simulink model "RIP_LQR_OK"  (Simulink 8.1)
settings: Solver=ode45  StartTime=0.0  StopTime=30  RelTol=1e-3
StopFcn:
  | plot(Data.time, Data.signals(1,1).values,'-r', 'LineWidth', 1.5)
  | hold on;
  | plot(Data.time, Data.signals(1,2).values,'-b', 'LineWidth',1.5)
  | grid;
  | legend('alpha','theta');
  | 
  | ylabel('alpha, theta [deg]');
libraries: aerolibconvert2 x4
settings Model: Creator=ThanhNhan  LastModifiedBy=ThanhNhan
settings DataIOCC: SignalLoggingSaveFormat=Dataset
settings OptimizationCC: ExpressionDepthLimit=128
settings DebuggingCC: FcnCallInpInsideContextMsg=EnableAllAsError
settings GRTTargetCC: CombineOutputUpdateFcns=on  GRTInterface=off

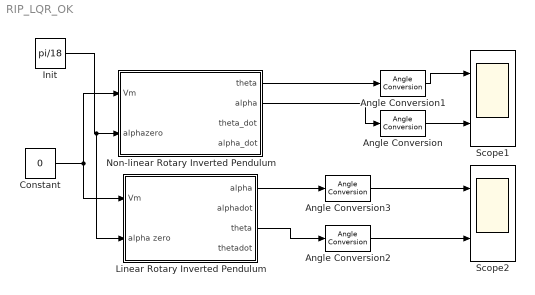
== system RIP_LQR_OK ==
  Angle Conversion{,1..3} (4 alike) : aerolibconvert2/Angle Conversion  IU=rad  OU=deg
  Constant : Constant  Value=0
  Init : Constant  Value=pi/18
  Linear Rotary Inverted Pendulum : Subsystem  mask{Jeq=0.004036, g=9.81, m=0.05562, L=0.1254, r=0.1095, Beq=0.0444, eta=0.69, Km=0.084026, Kt=0.084039, Rm=2.6, Jm=0.01}
      mask prompts: Jeq "Momen quan tinh tuong duong (Jeq)"; g "Gia toc trong truong (g)"; m "Khoi luong con lac (m)"; L "Nua chieu dai con lac (L)"; r "Nua chieu dai canh tay (r)"; Beq "He so can tuong duong (Beq)"; eta "Hieu suat dong co (eta)"; Km "Hang so suc dien dong (Km)"; Kt "Hang so momen (Kt)"; Rm "Dien tro phan ung (Rm)"; Jm "Momen quan tinh DC (Jm)"
  Non-linear Rotary Inverted Pendulum : Subsystem  mask{Jeq=0.004036, g=9.81, m=0.05562, L=0.1254, r=0.1095, Beq=0.0444, eta=0.69, Km=0.084026, Kt=0.084039, Rm=2.6, Jm=0.001}
      mask prompts: Jeq "Momen quán tính tuong duong (Jeq)"; g "Gia toc trong truong (g)"; m "Khoi luong con lac (m)"; L "Nua chieu dai con lac (L)"; r "Nua chieu dài cánh tay (r)"; Beq "He so can tuong duong (Beq)"; eta "Hieu suat dong co (eta)"; Km "Hang so suc dien dong (Km)"; Kt "Hang so momen  (Kt)"; Rm "Dien tro phan ung (Rm)"; Jm "Momen quan tinh dong co (Jm)"
  Scope1 : Scope  NumInputPorts=2
      settings: YMin=-9e+08~4.7025  YMax=-3.5e+08~4.72  SaveName=Data  SampleInput=on
  Scope2 : Scope  NumInputPorts=2
      settings: YMin=-9e+08~4.7025  YMax=-3.5e+08~4.72  SaveName=Data1  SampleInput=on
  wires:
  Constant/1 -> Non-linear Rotary Inverted Pendulum/1(Vm), Linear Rotary Inverted Pendulum/1(Vm)
  Init/1 -> Linear Rotary Inverted Pendulum/2(alpha zero), Non-linear Rotary Inverted Pendulum/2(alphazero)
  Non-linear Rotary Inverted Pendulum/1(theta) -> Angle Conversion1/1
  Angle Conversion/1 -> Scope1/2
  Angle Conversion1/1 -> Scope1/1
  Non-linear Rotary Inverted Pendulum/2(alpha) -> Angle Conversion/1
  Linear Rotary Inverted Pendulum/1(alpha) -> Angle Conversion3/1
  Angle Conversion2/1 -> Scope2/2
  Angle Conversion3/1 -> Scope2/1
  Linear Rotary Inverted Pendulum/3(theta) -> Angle Conversion2/1

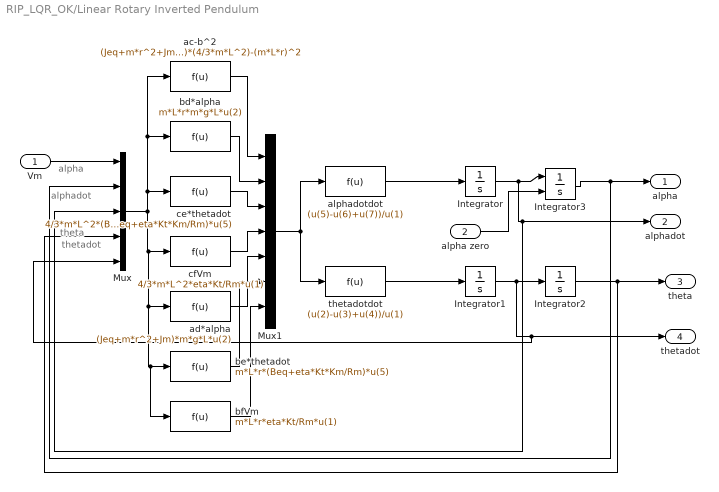
== system RIP_LQR_OK/Linear Rotary Inverted Pendulum ==
  note: thetadot
  note: theta
  note: alphadot
  note: alpha
  Vm : Inport
  alpha zero : Inport  Port=2
  Integrator : Integrator
  Integrator1 : Integrator
  Integrator2 : Integrator
  Integrator3 : Integrator  InitialConditionSource=external
  Mux : Mux  Inputs=5
  Mux1 : Mux  Inputs=7
  ac-b^2 : Fcn  Expr=(Jeq+m*r^2+Jm)*(4/3*m*L^2)-(m*L*r)^2
  ad*alpha : Fcn  Expr=(Jeq+m*r^2+Jm)*m*g*L*u(2)
  alphadotdot : Fcn  Expr=(u(5)-u(6)+u(7))/u(1)
  bd*alpha : Fcn  Expr=m*L*r*m*g*L*u(2)
  be*thetadot : Fcn  Expr=m*L*r*(Beq+eta*Kt*Km/Rm)*u(5)
  bfVm : Fcn  Expr=m*L*r*eta*Kt/Rm*u(1)
  ce*thetadot : Fcn  Expr=4/3*m*L^2*(Beq+eta*Kt*Km/Rm)*u(5)
  cfVm : Fcn  Expr=4/3*m*L^2*eta*Kt/Rm*u(1)
  thetadotdot : Fcn  Expr=(u(2)-u(3)+u(4))/u(1)
  alpha : Outport
  alphadot : Outport  Port=2
  theta : Outport  Port=3
  thetadot : Outport  Port=4
  wires:
  Vm/1 -> Mux/1
  Integrator/1 -> Mux/3, alphadot/1, Integrator3/1
  Integrator1/1 -> Mux/5, thetadot/1, Integrator2/1
  Mux1/1 -> thetadotdot/1, alphadotdot/1
  alphadotdot/1 -> Integrator/1
  thetadotdot/1 -> Integrator1/1
  Integrator3/1 -> Mux/2, alpha/1
  Integrator2/1 -> Mux/4, theta/1
  ac-b^2/1 -> Mux1/1
  bd*alpha/1 -> Mux1/2
  ce*thetadot/1 -> Mux1/3
  cfVm/1 -> Mux1/4
  ad*alpha/1 -> Mux1/5
  be*thetadot/1 -> Mux1/6
  bfVm/1 -> Mux1/7
  Mux/1 -> bfVm/1, be*thetadot/1, ad*alpha/1, cfVm/1, bd*alpha/1, ac-b^2/1, ce*thetadot/1
  alpha zero/1 -> Integrator3/2

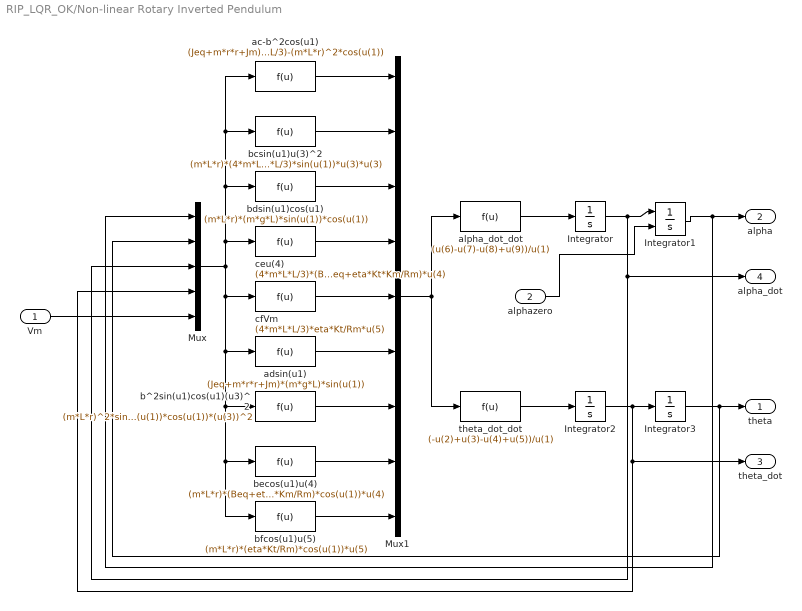
== system RIP_LQR_OK/Non-linear Rotary Inverted Pendulum ==
  Vm : Inport
  alphazero : Inport  Port=2
  Integrator : Integrator  UpperSaturationLimit=pi/18  LowerSaturationLimit=-pi/18
  Integrator1 : Integrator  InitialConditionSource=external  UpperSaturationLimit=pi/18  LowerSaturationLimit=-pi/18
  Integrator2 : Integrator
  Integrator3 : Integrator  UpperSaturationLimit=2  LowerSaturationLimit=-2
  Mux : Mux  Inputs=5
  Mux1 : Mux  Inputs=9
  ac-b^2cos(u1) : Fcn  Expr=(Jeq+m*r*r+Jm)*(4*m*L*L/3)-(m*L*r)^2*cos(u(1))
  adsin(u1) : Fcn  Expr=(Jeq+m*r*r+Jm)*(m*g*L)*sin(u(1))
  alpha_dot_dot : Fcn  Expr=(u(6)-u(7)-u(8)+u(9))/u(1)
  b^2sin(u1)cos(u1)(u3)^2 : Fcn  Expr=(m*L*r)^2*sin(u(1))*cos(u(1))*(u(3))^2
  bcsin(u1)u(3)^2 : Fcn  Expr=(m*L*r)*(4*m*L*L/3)*sin(u(1))*u(3)*u(3)
  bdsin(u1)cos(u1) : Fcn  Expr=(m*L*r)*(m*g*L)*sin(u(1))*cos(u(1))
  becos(u1)u(4) : Fcn  Expr=(m*L*r)*(Beq+eta*Kt*Km/Rm)*cos(u(1))*u(4)
  bfcos(u1)u(5) : Fcn  Expr=(m*L*r)*(eta*Kt/Rm)*cos(u(1))*u(5)
  ceu(4) : Fcn  Expr=(4*m*L*L/3)*(Beq+eta*Kt*Km/Rm)*u(4)
  cfVm : Fcn  Expr=(4*m*L*L/3)*eta*Kt/Rm*u(5)
  theta_dot_dot : Fcn  Expr=(-u(2)+u(3)-u(4)+u(5))/u(1)
  theta : Outport
  alpha : Outport  Port=2
  theta_dot : Outport  Port=3
  alpha_dot : Outport  Port=4
  wires:
  alpha_dot_dot/1 -> Integrator/1
  Integrator/1 -> Mux/3, alpha_dot/1, Integrator1/1
  theta_dot_dot/1 -> Integrator2/1
  Integrator1/1 -> Mux/1, alpha/1
  Integrator3/1 -> Mux/2, theta/1
  ac-b^2cos(u1)/1 -> Mux1/1
  bcsin(u1)u(3)^2/1 -> Mux1/2
  bdsin(u1)cos(u1)/1 -> Mux1/3
  ceu(4)/1 -> Mux1/4
  cfVm/1 -> Mux1/5
  adsin(u1)/1 -> Mux1/6
  b^2sin(u1)cos(u1)(u3)^2/1 -> Mux1/7
  becos(u1)u(4)/1 -> Mux1/8
  bfcos(u1)u(5)/1 -> Mux1/9
  Mux1/1 -> theta_dot_dot/1, alpha_dot_dot/1
  Mux/1 -> ceu(4)/1, bdsin(u1)cos(u1)/1, bcsin(u1)u(3)^2/1, ac-b^2cos(u1)/1, bfcos(u1)u(5)/1, becos(u1)u(4)/1, b^2sin(u1)cos(u1)(u3)^2/1, adsin(u1)/1, cfVm/1
  Integrator2/1 -> Mux/4, theta_dot/1, Integrator3/1
  Vm/1 -> Mux/5
  alphazero/1 -> Integrator1/2
